simulink model "Main_Sim"  (R2018b)
settings: Solver=VariableStepAuto  StartTime=0.0  StopTime=500.0  RelTol=1e-3  EnableMultiTasking=on
undefined symbols (not defined in the file): qd
libraries: PD_Controller_Lib x1, Satellite_Dynamics x1
settings Model: Creator=devantormey  LastModifiedBy=devantormey
settings OptimizationCC: LifeSpan=inf
settings DebuggingCC: SFUnexpectedBacktrackingDiag=warning  SFNoUnconditionalDefaultTransitionDiag=warning
settings SFSimCC: SimUseLocalCustomCode=off
settings RTWCC: RTWUseLocalCustomCode=off
settings CodeAppCC: StateflowObjectComments=on
settings GRTTargetCC: TargetLangStandard=C89/C90 (ANSI)  GeneratePreprocessorConditionals=Disable all
settings ConfigComp: CovMetricSettings=dw  CovHtmlReporting=on  CovSaveCumulativeToWorkspaceVar=on  CovSaveSingleToWorkspaceVar=on  CovExternalEMLEnable=off

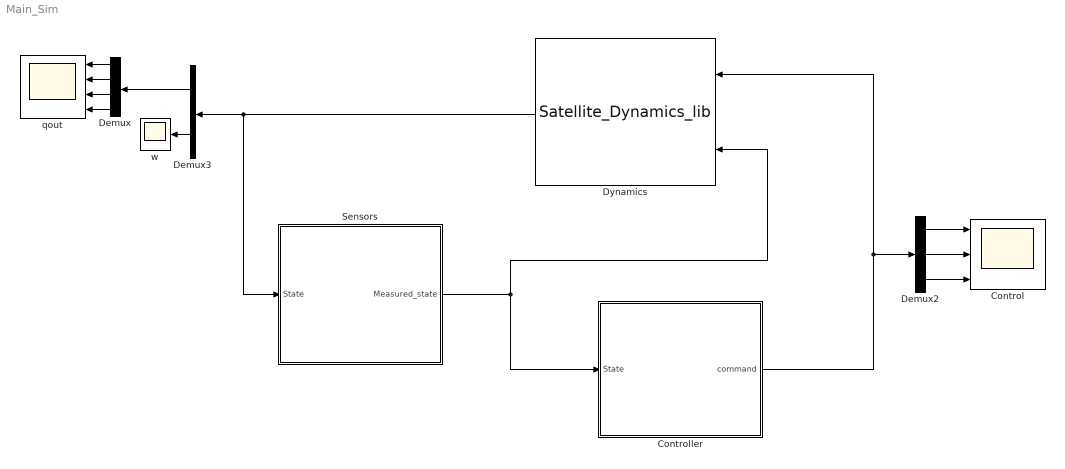
== system Main_Sim ==
  Control : Scope  NumInputPorts=3
  Controller : Subsystem
  Demux : Demux
  Demux2 : Demux  Outputs=3
  Demux3 : Demux  Outputs=[4 3]
  "Dynamics " : Satellite_Dynamics/Satellite_Dynamics_lib  SystemSampleTime=-1
      link override Constant: Value=J
  Sensors : Subsystem
  qout : Scope  NumInputPorts=4
  w : Scope
  wires:
  Demux/1 -> qout/1
  Demux/2 -> qout/2
  Demux/3 -> qout/3
  Demux/4 -> qout/4
  Demux2/2 -> Control/2
  Demux2/1 -> Control/1
  Demux2/3 -> Control/3
  Demux3/1 -> Demux/1
  Demux3/2 -> w/1
  Controller/1(command) -> Demux2/1, "Dynamics "/1
  Sensors/1(Measured_state) -> Controller/1(State), "Dynamics "/2
  "Dynamics "/1 -> Sensors/1(State), Demux3/1

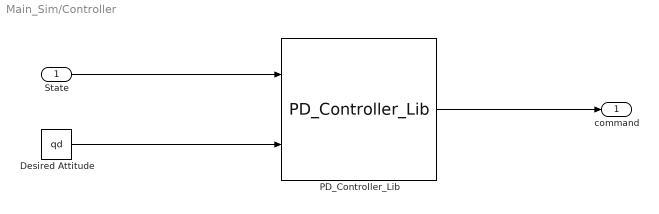
== system Main_Sim/Controller ==
  State : Inport
  Desired Attitude : Constant  Value=qd
  PD_Controller_Lib : PD_Controller_Lib/PD_Controller_Lib  SystemSampleTime=-1
  command : Outport
  wires:
  PD_Controller_Lib/1 -> command/1
  State/1 -> PD_Controller_Lib/1
  Desired Attitude/1 -> PD_Controller_Lib/2

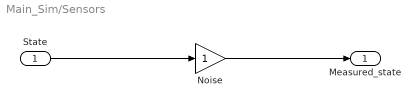
== system Main_Sim/Sensors ==
  State : Inport
  Noise : Gain
  Measured_state : Outport
  wires:
  State/1 -> Noise/1
  Noise/1 -> Measured_state/1
